simulink model "vel_ctrl"  (R2022a)
settings: Solver=VariableStepAuto  StartTime=0.0  StopTime=10  RelTol=1e-3
settings Model: Creator=abiyyumufti  LastModifiedBy=abiyyumufti

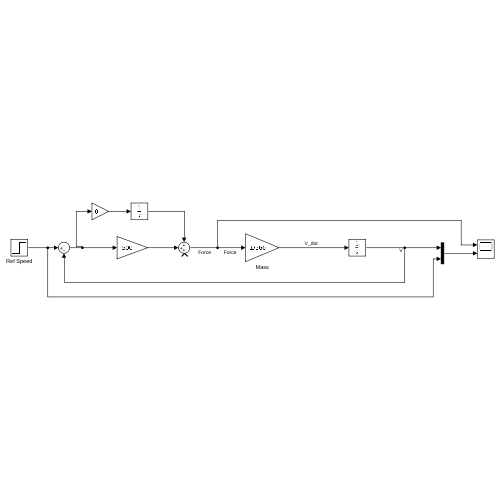
[thumbnail: Simulink's stored preview of the top-level diagram]
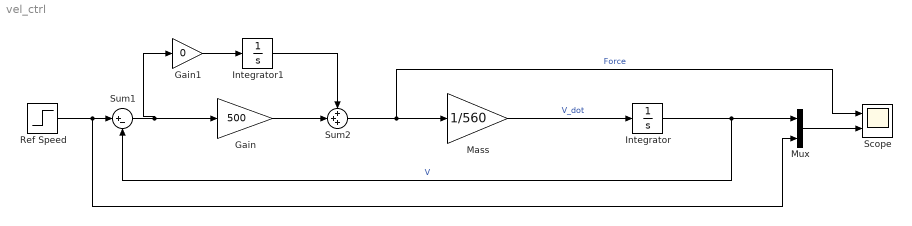
== system vel_ctrl ==
  Gain : Gain  Gain=500
  Gain1 : Gain  Gain=0
  Integrator : Integrator
  Integrator1 : Integrator
  Mass : Gain  Gain=1/560
  Mux : Mux  Inputs=2
  Ref Speed : Step  Time=0  After=250  SampleTime=0
  Scope : Scope  NumInputPorts=2
  Sum1 : Sum  Inputs=|+-
  Sum2 : Sum  Inputs=+++
  wires:
  Sum2/1 -> Scope/1, Mass/1  "Force"
  Mass/1 -> Integrator/1  "V_dot"
  Integrator/1 -> Sum1/2, Mux/1  "V"
  Ref Speed/1 -> Mux/2, Sum1/1
  Sum1/1 -> Gain1/1, Gain/1
  Mux/1 -> Scope/2
  Gain1/1 -> Integrator1/1
  Gain/1 -> Sum2/2
  Integrator1/1 -> Sum2/1
